simulink model "test_bus_selector"  (R2018a)
settings: Solver=VariableStepAuto  StartTime=0.0  StopTime=10.0  RelTol=1e-3
settings Model: Creator=HIL105  LastModifiedBy=HIL105

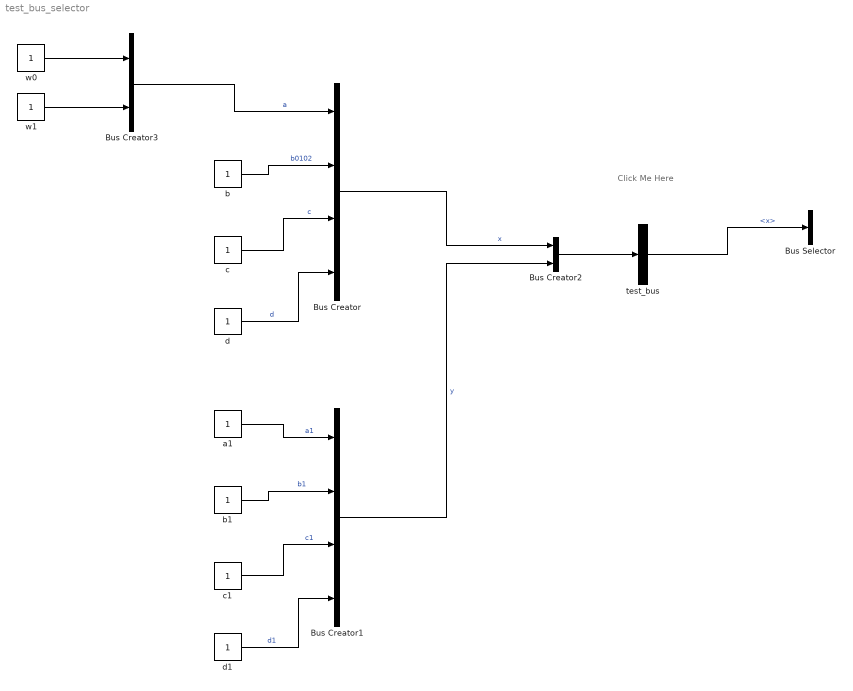
== system test_bus_selector ==
  note: Click Me Here
  Bus Creator : BusCreator  Inputs=4
  Bus Creator1 : BusCreator  Inputs=4
  Bus Creator2 : BusCreator  Inputs=2
  Bus Creator3 : BusCreator  Inputs=2
  Bus Selector : BusSelector  OutputSignals=a,b0102,c,d
  a1 : Constant
  b : Constant
  b1 : Constant
  c : Constant
  c1 : Constant
  d : Constant
  d1 : Constant
  test_bus : BusSelector  OutputSignals=x
  w0 : Constant
  w1 : Constant
  wires:
  b/1 -> Bus Creator/2  "b0102"
  Bus Creator3/1 -> Bus Creator/1  "a"
  c/1 -> Bus Creator/3  "c"
  d/1 -> Bus Creator/4  "d"
  d1/1 -> Bus Creator1/4  "d1"
  c1/1 -> Bus Creator1/3  "c1"
  a1/1 -> Bus Creator1/1  "a1"
  b1/1 -> Bus Creator1/2  "b1"
  Bus Creator/1 -> Bus Creator2/1  "x"
  Bus Creator1/1 -> Bus Creator2/2  "y"
  Bus Creator2/1 -> test_bus/1
  w0/1 -> Bus Creator3/1
  w1/1 -> Bus Creator3/2
  test_bus/1 -> Bus Selector/1  "<x>"
